simulink model "RFpracticeReflectedPower"  (R2022b)
settings: Solver=VariableStepAuto  StartTime=0.0  StopTime=10.0  RelTol=1e-3
libraries: simrfV2util1 x6, simrfV2sources1 x4, simrfV2junction1 x1, simrfV2elements x1
settings Model: Creator=Joseph  LastModifiedBy=Joseph

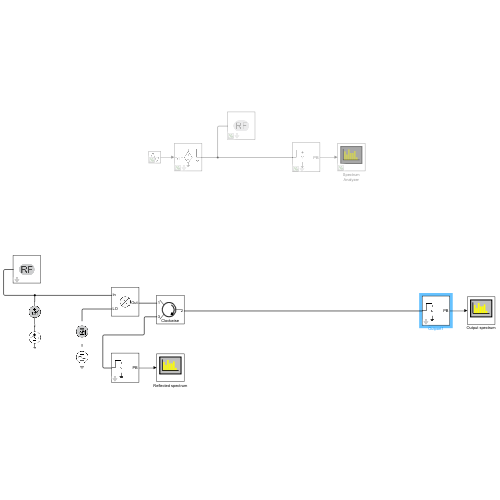
[thumbnail: Simulink's stored preview of the top-level diagram]
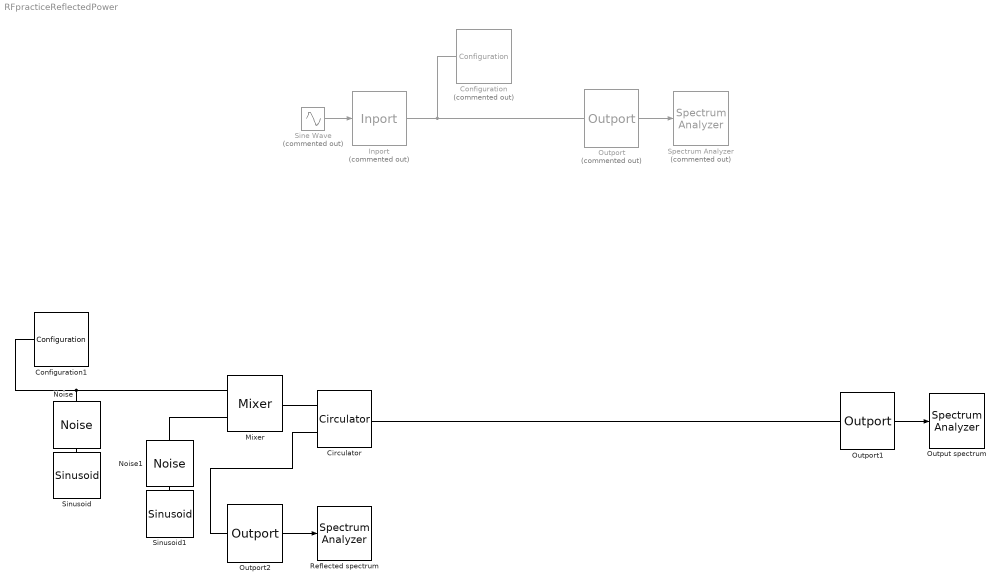
== system RFpracticeReflectedPower ==
  Circulator : simrfV2junction1/Circulator  classname=circulators  DataSource=Network-parameters  NumPorts=3  DeviceCirculator=Circulator clockwise  DeviceDivider=T power divider  DeviceCoupler=Directional coupler  Paramtype=S-parameters  Sparam=[0 0 1; 1 0 0; 0 1 0]  SparamFreq=1e9 Hz  SparamZ0=50  Phase12=0  Phase33=0  Alpha=0  NumberDividerOutports=2  Coupling=0  Directivity=inf  InsertionLoss=inf  ReturnLoss=inf  InternalGrounding=on  SparamRepresentation=Frequency domain  FitOpt=Share all poles  FitTol=-40  MaxPoles=48
  Configuration : simrfV2util1/Configuration  Commented=on  AutoFreq=on  Tones=[0] Hz  Harmonics=[1]  NormalizeCarrierPower=on  SolverType=Auto  UseCCode=on  StepSize=1e-6 s  AddNoise=on  defaultRNG=on  Seed=0  Temperature=290.0 K  SolverDelFlag=0  AbsTol=1e-6  RelTol=1e-3  MaxIter=10  ErrorEstimationType=2-norm over all variables  EnableInterpFilter=on  HiddenFIRfilterControllerParam=on  SmallSignalApprox=off  AllSimFreqs=on  SimFreqs=[] Hz  SimFreqsInternal=[]  SamplesPerFrame=1
  Configuration1 : simrfV2util1/Configuration  AutoFreq=on  Tones=[0] Hz  Harmonics=[1]  NormalizeCarrierPower=on  SolverType=Auto  UseCCode=on  StepSize=1e-9 s  AddNoise=on  defaultRNG=on  Seed=0  Temperature=290.0 K  SolverDelFlag=0  AbsTol=1e-6  RelTol=1e-3  MaxIter=10  ErrorEstimationType=2-norm over all variables  EnableInterpFilter=on  HiddenFIRfilterControllerParam=off  SmallSignalApprox=off  AllSimFreqs=on  SimFreqs=[] Hz  SimFreqsInternal=[]  SamplesPerFrame=1
  Inport : simrfV2util1/Inport  Commented=on  SimulinkInputSignalType=Ideal voltage  CarrierFreq=0 kHz  ZS=0  UseSqWave=off  NumCoeff=10  Bias=0  DutyCyc=50  InternalGrounding=on
  Mixer : simrfV2elements/Mixer  classname=mixer  Source_linear_gain=Available power gain  linear_gain=0 dB  Zin=50  Zout=50  ZLO=inf  Source_Poly=Even and odd order  Poly_Coeffs=[0 1]  IPType=Output  IP2=Inf dBm  IP3=Inf dBm  P1dB=Inf dBm  Psat=Inf dBm  Gcomp=Inf dBm  NF=0  InternalGrounding=on
  Noise : simrfV2sources1/Noise  SimulinkInputSignalType=Ideal voltage  NoiseType=White  NoisePSD=5e-15  CarrierFreq=0 Hz  AutoImpulseLength=on  ImpulseLength=1e-10 s  InternalGrounding=off
  Noise1 : simrfV2sources1/Noise  SimulinkInputSignalType=Ideal voltage  NoiseType=White  NoisePSD=5e-15  CarrierFreq=0 Hz  AutoImpulseLength=on  ImpulseLength=1e-10 s  InternalGrounding=off
  Outport : simrfV2util1/Outport  Commented=on  SensorType=Ideal voltage  OutputFormat=Real Passband  CarrierFreq=0 kHz  ZL=Inf  InternalGrounding=on  StepSize=0.000125 s  AutoStep=on
  Outport1 : simrfV2util1/Outport  SensorType=Ideal voltage  OutputFormat=Real Passband  CarrierFreq=0 kHz  ZL=Inf  InternalGrounding=on  StepSize=0.000125 s  AutoStep=on
  Outport2 : simrfV2util1/Outport  SensorType=Ideal voltage  OutputFormat=Real Passband  CarrierFreq=0 kHz  ZL=Inf  InternalGrounding=on  StepSize=0.000125 s  AutoStep=on
  Output spectrum : SpectrumAnalyzer  Tag=simrfV2util1/Spectrum Analyzer
  Reflected spectrum : SpectrumAnalyzer  Tag=simrfV2util1/Spectrum Analyzer
  Sine Wave : Sin  Commented=on  Frequency=2*pi*1000  SampleTime=0
  Sinusoid : simrfV2sources1/Sinusoid  SineSourceType=Ideal voltage  VO_I=0 V  IO_I=0 A  VO_Q=0 V  IO_Q=0 A  VA_I=1 V  IA_I=0 A  VA_Q=0 V  IA_Q=0 A  Fmod=100 MHz  TD=0 s  CarrierFreq=0 Hz  InternalGrounding=on
  Sinusoid1 : simrfV2sources1/Sinusoid  SineSourceType=Ideal voltage  VO_I=0 V  IO_I=0 A  VO_Q=0 V  IO_Q=0 A  VA_I=1 V  IA_I=0 A  VA_Q=0 V  IA_Q=0 A  Fmod=99 MHz  TD=0 s  CarrierFreq=0 Hz  InternalGrounding=on
  Spectrum Analyzer : SpectrumAnalyzer  Tag=simrfV2util1/Spectrum Analyzer  Commented=on
  wires:
  Outport/1 -> Spectrum Analyzer/1
  Sine Wave/1 -> Inport/1
  Outport1/1 -> Output spectrum/1
  Outport2/1 -> Reflected spectrum/1
  connections:
  Outport/LConn1 -- Configuration/LConn1 -- Inport/RConn1
  Configuration1/LConn1 -- Mixer/LConn1 -- Noise/LConn1
  Sinusoid/LConn1 -- Noise/RConn1
  Sinusoid1/LConn1 -- Noise1/RConn1
  Noise1/LConn1 -- Mixer/LConn2
  Circulator/LConn1 -- Mixer/RConn1
  Outport2/LConn1 -- Circulator/LConn2
  Outport1/LConn1 -- Circulator/RConn1
